simulink model "20240109_HVDCMMCInterconnection"  (R2023b)
settings: Solver=FixedStepDiscrete  StartTime=0.0  StopTime=2  FixedStep=Ts_Power  RelTol=1e-4  EnableMultiTasking=on
PreLoadFcn:
  | HVDCMMCInterconnectionParam
StartFcn:
  | tic
StopFcn:
  | toc
values from neighbouring files (symbols this model uses):
  C_PM = 1.758e-3    (= 0.001758)    [HVDCMMCInterconnectionParam.m]
  Cg = 50e-9    (= 5e-08)    [HVDCMMCInterconnectionParam.m]
  D_R = 0.001    [HVDCMMCInterconnectionParam.m]
  D_Rs = 1e8    (= 100000000)    [HVDCMMCInterconnectionParam.m]
  D_Vf = 0    [HVDCMMCInterconnectionParam.m]
  Fnom = 50    [HVDCMMCInterconnectionParam.m]
  HRM = 2    [HVDCMMCInterconnectionParam.m]
  Ki_Ireg = 6    [HVDCMMCInterconnectionParam.m]
  Ki_Preg = 1.0    (= 1)    [HVDCMMCInterconnectionParam.m]
  Ki_Qreg = 1.0    (= 1)    [HVDCMMCInterconnectionParam.m]
  Ki_VDCreg = 100    [HVDCMMCInterconnectionParam.m]
  Kp_Ireg = 0.6    [HVDCMMCInterconnectionParam.m]
  Kp_Preg = 0.5/3    (= 0.166666666667)    [HVDCMMCInterconnectionParam.m]
  Kp_Qreg = 0.5/3    (= 0.166666666667)    [HVDCMMCInterconnectionParam.m]
  Kp_VDCreg = 4    [HVDCMMCInterconnectionParam.m]
  L_cable = 15e-3    (= 0.015)    [HVDCMMCInterconnectionParam.m]
  Larm = Larm_pu*(Zb_ac/(2*pi*Fnom))    [HVDCMMCInterconnectionParam.m]
  Lff = Larm_pu/2    (= 0.075)    [HVDCMMCInterconnectionParam.m]
  Limits_Ireg = [ 2.0  -2.0]    [HVDCMMCInterconnectionParam.m]
  Limits_Preg = [ 1.2, 0.8 ]    [HVDCMMCInterconnectionParam.m]
  Limits_Qreg = [ 0.25, -0.25 ]    [HVDCMMCInterconnectionParam.m]
  Limits_VDCreg = [ 2.0  -2.0]    [HVDCMMCInterconnectionParam.m]
  Lxfo = 0.12    [HVDCMMCInterconnectionParam.m]
  Nb_PM = 36    [HVDCMMCInterconnectionParam.m]
  Pnom = 1000e6    (= 1000000000)    [HVDCMMCInterconnectionParam.m]
  R_cable = 0.5    [HVDCMMCInterconnectionParam.m]
  R_startup = 400    [HVDCMMCInterconnectionParam.m]
  Rarm = Rarm_pu*Zb_ac    [HVDCMMCInterconnectionParam.m]
  Rff = Rarm_pu/2    (= 0.00075)    [HVDCMMCInterconnectionParam.m]
  Rg = 100    [HVDCMMCInterconnectionParam.m]
  Rxfo = 0.003    [HVDCMMCInterconnectionParam.m]
  Slope_Pref = 0.5    [HVDCMMCInterconnectionParam.m]
  Slope_Qref = 0.5    [HVDCMMCInterconnectionParam.m]
  Slope_Vdc_ref = Vnom_dc/5    (= 128000)    [HVDCMMCInterconnectionParam.m]
  Tbrk1_On = 0.1    [HVDCMMCInterconnectionParam.m]
  Tbrk2_On = 1.0    (= 1)    [HVDCMMCInterconnectionParam.m]
  Tdeblock = 1.5    [HVDCMMCInterconnectionParam.m]
  Tfault = 9999    [HVDCMMCInterconnectionParam.m]
  Ton_Converter2 = 4    [HVDCMMCInterconnectionParam.m]
  Ton_PQreg = 4    [HVDCMMCInterconnectionParam.m]
  Ton_VDCreg = 1.5    [HVDCMMCInterconnectionParam.m]
  Ts = Ts_Control    (= 4e-05)    [HVDCMMCInterconnectionParam.m]
  Ts_Control = 40e-6    (= 4e-05)    [HVDCMMCInterconnectionParam.m]
  Ts_Power = 20e-6    (= 2e-05)    [HVDCMMCInterconnectionParam.m]
  Vb_ac = sqrt(2/3)*Vnom_sec    [HVDCMMCInterconnectionParam.m]
  Vb_dc = Vnom_dc    (= 640000)    [HVDCMMCInterconnectionParam.m]
  Vc0_PM = 0    [HVDCMMCInterconnectionParam.m]
  Vnom_dc = 640e3    (= 640000)    [HVDCMMCInterconnectionParam.m]
  Vnom_prim = 400e3    (= 400000)    [HVDCMMCInterconnectionParam.m]
  Vnom_sec = 333e3    (= 333000)    [HVDCMMCInterconnectionParam.m]
  w = 2*pi*Fnom    (= 314.159265359)    [HVDCMMCInterconnectionParam.m]
undefined symbols (not defined in the file or in its folder): DiscIntNeverNeededParam, gcbh, Pcc, S, sps_AC, sps_ACDC2, sps_rtmsupport
libraries: simulink x48, spsControlledVoltageSourceLib x30, spsCurrentMeasurementLib x30, MMC_Lib x30, spsDiodeLib x20, spsSeriesRLCBranchLib x14, powerlib_extras x12, spsVoltageMeasurementLib x12, spsSecondOrderFilterLib x8, spsabctodq0Lib x8, spsGroundLib x7, spsMeanLib x4
(part 8 of 9)

== system 20240109_HVDCMMCInterconnection/MMC/Half-Bridge MMC Ap (Aggregate model of 36 PM)7 ==
  Uref : Inport
  Controlled Voltage Source : spsControlledVoltageSourceLib/Controlled Voltage Source  Initialize=on  Source_Type=AC  Amplitude=0  Phase=0  Frequency=0  Measurements=None
  Controlled Voltage Source1 : spsControlledVoltageSourceLib/Controlled Voltage Source  Initialize=on  Source_Type=AC  Amplitude=0  Phase=0  Frequency=0  Measurements=None
  Current Measurement : spsCurrentMeasurementLib/Current Measurement  PhasorSimulation=off  OutputType=Complex  PSBequivalent=0
  Current Measurement1 : spsCurrentMeasurementLib/Current Measurement  PhasorSimulation=off  OutputType=Complex  PSBequivalent=0
  Demux : Demux  Outputs=2
  Diode : spsDiodeLib/Diode  Ron=Ron_Diode  Lon=0  Vf=Vf_Diode  IC=0  UseSnubber=0  Rs=Rs_Diode  Cs=Cs_Diode  Measurements=off
  Diode1 : spsDiodeLib/Diode  Ron=Ron_Diode  Lon=0  Vf=Vf_Diode  IC=0  UseSnubber=0  Rs=Rs_Diode  Cs=Cs_Diode  Measurements=off
  Discrete-Time Integrator1 : DiscreteIntegrator  IntegratorMethod=Integration: Trapezoidal  gainval=1  InitialCondition=Vc_Initial  SampleTime=Ts  UpperSaturationLimit=5000  LowerSaturationLimit=500  ICPrevOutput=DiscIntNeverNeededParam  ICPrevScaledInput=DiscIntNeverNeededParam
  Gain1 : Gain  Gain=n
  Gain4 : Gain  Gain=1/(C*n)
  Gain5 : Gain  Gain=2
  Mux1 : Mux  Inputs=2
  Product3 : Product
  Product4 : Product
  Scope : Scope  NumInputPorts=3
  Sum3 : Sum  Inputs=1  InputSameDT=on  SaturateOnIntegerOverflow=on  OutDataTypeStr=Inherit: Same as first input
  Sum4 : Sum  Inputs=+-  InputSameDT=on  SaturateOnIntegerOverflow=on  OutDataTypeStr=Inherit: Same as first input
  Unit Delay2 : UnitDelay  SampleTime=Ts  HasFrameUpgradeWarning=on
  Unit Delay5 : UnitDelay  InitialCondition=Vc_Initial  SampleTime=Ts  HasFrameUpgradeWarning=on
  Unit Delay6 : UnitDelay  InitialCondition=Vc_Initial  SampleTime=Ts  HasFrameUpgradeWarning=on
  Voltage Measurement : spsVoltageMeasurementLib/Voltage Measurement  PhasorSimulation=off  OutputType=Complex  PSBequivalent=0
  1 : PMIOPort  Side=Left
  2 : PMIOPort  Port=2  Side=Left
  Vc : Outport  VectorParamsAs1DForOutWhenUnconnected=off
  wires:
  Demux/1 -> Scope/1, [Vin]
  [Vin] -> Controlled Voltage Source/1
  Current Measurement1/1 -> [Icap]
  Product3/1 -> Sum3/1
  Demux/2 -> Scope/2, [Vbl]
  [Imod] -> Mux1/1
  Sum3/1 -> Gain4/1
  Unit Delay5/1 -> Sum4/2
  Gain5/1 -> Sum4/1
  Mux1/1 -> Unit Delay2/1
  Uref/1 -> Gain1/1
  Sum4/1 -> Vc/1, Product4/2
  Current Measurement/1 -> [Imod]
  Unit Delay2/1 -> Product3/2
  Discrete-Time Integrator1/1 -> Unit Delay6/1
  Product4/1 -> Demux/1
  [Vbl] -> Controlled Voltage Source1/1
  [Icap] -> Mux1/2
  Gain4/1 -> Discrete-Time Integrator1/1
  Unit Delay6/1 -> Gain5/1, Unit Delay5/1
  Gain1/1 -> Product3/1, Product4/1
  Voltage Measurement/1 -> [Vsm]
  [Vsm] -> Scope/3
  connections:
  Diode1/LConn1 -- Current Measurement/RConn1 -- Diode/RConn1
  Controlled Voltage Source1/LConn1 -- Diode/LConn1 -- 2/RConn1 -- Voltage Measurement/LConn2
  Controlled Voltage Source1/RConn1 -- Current Measurement1/RConn1
  Diode1/RConn1 -- Current Measurement1/LConn1
  Controlled Voltage Source/RConn1 -- 1/RConn1 -- Voltage Measurement/LConn1
  Controlled Voltage Source/LConn1 -- Current Measurement/LConn1

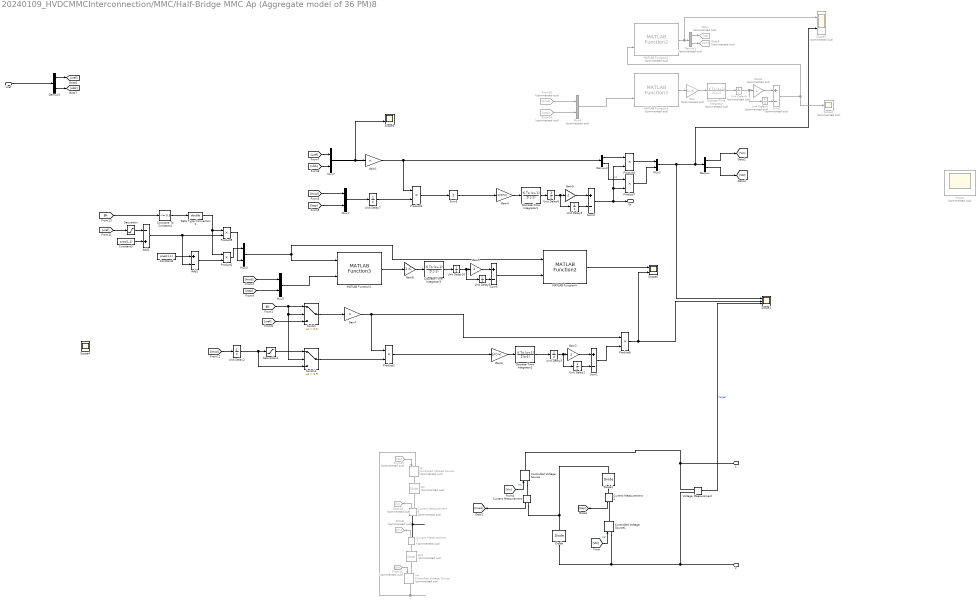
== system 20240109_HVDCMMCInterconnection/MMC/Half-Bridge MMC Ap (Aggregate model of 36 PM)8 ==
  Uref : Inport
  Add1 : Sum  Inputs=+-
  Add2 : Sum  Inputs=-+
  Compare To Constant1 : simulink/Logic and Bit Operations/Compare To Constant  relop=<=  const=0.5  OutDataTypeStr=boolean
  Constant3 : Constant  Value=ones(1,1)
  Constant4 : Constant  Value=ones(1,1)
  Controlled Voltage Source : spsControlledVoltageSourceLib/Controlled Voltage Source  Initialize=on  Source_Type=AC  Amplitude=0  Phase=0  Frequency=0  Measurements=None
  Controlled Voltage Source1 : spsControlledVoltageSourceLib/Controlled Voltage Source  Initialize=on  Source_Type=AC  Amplitude=0  Phase=0  Frequency=0  Measurements=None
  Current Measurement : spsCurrentMeasurementLib/Current Measurement  PhasorSimulation=off  OutputType=Complex  PSBequivalent=0
  Current Measurement1 : spsCurrentMeasurementLib/Current Measurement  PhasorSimulation=off  OutputType=Complex  PSBequivalent=0
  Current Measurement7 : spsCurrentMeasurementLib/Current Measurement  Commented=on  PhasorSimulation=off  OutputType=Complex  PSBequivalent=0
  Current Measurement8 : spsCurrentMeasurementLib/Current Measurement  Commented=on  PhasorSimulation=off  OutputType=Complex  PSBequivalent=0
  Data Type Conversion2 : DataTypeConversion  OutDataTypeStr=double  SaturateOnIntegerOverflow=off  RndMeth=Floor
  Demux : Demux  Outputs=2
  Demux1 : Demux  Commented=on  Outputs=2
  Demux2 : Demux  Outputs=2
  Demux5 : Demux  Outputs=2
  Diode : spsDiodeLib/Diode  Ron=0.0001  Lon=0  Vf=0.0001  IC=0  UseSnubber=0  Rs=1e9  Cs=Cs_Diode  Measurements=off
  Diode1 : spsDiodeLib/Diode  Ron=0.0001  Lon=0  Vf=0.0001  IC=0  UseSnubber=0  Rs=1e9  Cs=Cs_Diode  Measurements=off
  Discrete-Time Integrator : DiscreteIntegrator  Commented=on  IntegratorMethod=Integration: Trapezoidal  gainval=1  InitialCondition=Vc_Initial  SampleTime=Ts  UpperSaturationLimit=5000  LowerSaturationLimit=500  ICPrevOutput=DiscIntNeverNeededParam  ICPrevScaledInput=DiscIntNeverNeededParam
  Discrete-Time Integrator1 : DiscreteIntegrator  IntegratorMethod=Integration: Trapezoidal  gainval=1  InitialCondition=Vc_Initial  SampleTime=Ts  UpperSaturationLimit=5000  LowerSaturationLimit=500  ICPrevOutput=DiscIntNeverNeededParam  ICPrevScaledInput=DiscIntNeverNeededParam
  Discrete-Time Integrator2 : DiscreteIntegrator  IntegratorMethod=Integration: Trapezoidal  gainval=1  InitialCondition=Vc_Initial  SampleTime=Ts  UpperSaturationLimit=5000  LowerSaturationLimit=500  ICPrevOutput=DiscIntNeverNeededParam  ICPrevScaledInput=DiscIntNeverNeededParam
  Discrete-Time Integrator3 : DiscreteIntegrator  IntegratorMethod=Integration: Trapezoidal  gainval=1  InitialCondition=Vc_Initial  SampleTime=Ts  UpperSaturationLimit=5000  LowerSaturationLimit=500  ICPrevOutput=DiscIntNeverNeededParam  ICPrevScaledInput=DiscIntNeverNeededParam
  Dp : spsDiodeLib/Diode  Commented=on  Ron=Ron_Diode  Lon=0  Vf=Vf_Diode  IC=0  UseSnubber=off  Rs=Rs_Diode  Cs=Cs_Diode  Measurements=off
  Dp1 : spsDiodeLib/Diode  Commented=on  Ron=Ron_Diode  Lon=0  Vf=Vf_Diode  IC=0  UseSnubber=off  Rs=Rs_Diode  Cs=Cs_Diode  Measurements=off
  From10 : From  Commented=on  GotoTag=Imod
  From14 : From  Commented=on  GotoTag=Icap
  From15 : From  Commented=on  GotoTag=Vp
  From16 : From  Commented=on  GotoTag=Vm
  Gain : Gain  Commented=on  Gain=-1./C
  Gain1 : Gain  Gain=n
  Gain2 : Gain  Gain=2
  Gain3 : Gain  Gain=1/(C*n)
  Gain4 : Gain  Gain=1/(C*n)
  Gain5 : Gain  Gain=2
  Gain6 : Gain  Gain=-1./C
  Gain7 : Gain  Gain=n
  Gain8 : Gain  Commented=on  Gain=2
  Gain9 : Gain  Gain=2
  Goto : Goto  Commented=on  GotoTag=Vp
  Goto18 : Goto  Commented=on  GotoTag=Ip
  Goto5 : Goto  Commented=on  GotoTag=Vm
  Goto8 : Goto  Commented=on  GotoTag=Im
  MATLAB Function1 : spsHalfBridgeMMCmodel/AVG Discrete/MATLAB Function3  n=1  ModelType=3
  MATLAB Function2 : spsHalfBridgeMMCmodel/AVG Discrete/MATLAB Function2  Commented=on  n=1  ModelType=3
  MATLAB Function3 : spsHalfBridgeMMCmodel/AVG Discrete/MATLAB Function3  Commented=on  n=1  ModelType=3
  MATLAB Function4 : spsHalfBridgeMMCmodel/AVG Discrete/MATLAB Function2  n=1  ModelType=3
  Mux{1..3,5,7} (5 alike) : Mux  Inputs=2
  Mux4 : Mux  Commented=on  Inputs=2
  Product{1..5,7..8} (7 alike) : Product
  Saturation : Saturate  UpperLimit=1  LowerLimit=-1
  Saturation2 : Saturate  UpperLimit=inf  LowerLimit=0
  Scope : Scope  Commented=on  NumInputPorts=2
  Scope1 : Scope  NumInputPorts=3
  Scope2 : Scope  Commented=on
  Scope3 : Scope  Commented=on  NumInputPorts=2
  Scope4 : Scope  NumInputPorts=2
  Scope5 : Scope  NumInputPorts=2
  Scope6 : Scope  NumInputPorts=2
  Sum1 : Sum  Inputs=+-  InputSameDT=on  SaturateOnIntegerOverflow=on  OutDataTypeStr=Inherit: Same as first input
  Sum2 : Sum  Commented=on  Inputs=+-  InputSameDT=on  SaturateOnIntegerOverflow=on  OutDataTypeStr=Inherit: Same as first input
  Sum3 : Sum  Inputs=1  InputSameDT=on  SaturateOnIntegerOverflow=on  OutDataTypeStr=Inherit: Same as first input
  Sum4 : Sum  Inputs=+-  InputSameDT=on  SaturateOnIntegerOverflow=on  OutDataTypeStr=Inherit: Same as first input
  Sum5 : Sum  Inputs=+-  InputSameDT=on  SaturateOnIntegerOverflow=on  OutDataTypeStr=Inherit: Same as first input
  Switch : Switch  Criteria=u2 > Threshold  Threshold=0.5  SaturateOnIntegerOverflow=off  InputSameDT=off
  Switch1 : Switch  Criteria=u2 > Threshold  Threshold=0.5  SaturateOnIntegerOverflow=off  InputSameDT=off
  Unit Delay{1,3,5..6,9..10} (6 alike) : UnitDelay  InitialCondition=Vc_Initial  SampleTime=Ts  HasFrameUpgradeWarning=on
  Unit Delay2 : UnitDelay  SampleTime=Ts  HasFrameUpgradeWarning=on
  Unit Delay4 : UnitDelay  Commented=on  InitialCondition=Vc_Initial  SampleTime=Ts  HasFrameUpgradeWarning=on
  Unit Delay7 : UnitDelay  SampleTime=Ts  HasFrameUpgradeWarning=on
  Unit Delay8 : UnitDelay  Commented=on  InitialCondition=Vc_Initial  SampleTime=Ts  HasFrameUpgradeWarning=on
  Vm : spsControlledVoltageSourceLib/Controlled Voltage Source  Commented=on  Initialize=off  Source_Type=AC  Amplitude=0  Phase=0  Frequency=0  Measurements=None
  Voltage Measurement : spsVoltageMeasurementLib/Voltage Measurement  PhasorSimulation=off  OutputType=Complex  PSBequivalent=0
  Vp : spsControlledVoltageSourceLib/Controlled Voltage Source  Commented=on  Initialize=off  Source_Type=AC  Amplitude=0  Phase=0  Frequency=0  Measurements=None
  1 : PMIOPort  Side=Left
  2 : PMIOPort  Port=2  Side=Left
  Vc : Outport  VectorParamsAs1DForOutWhenUnconnected=off
  wires:
  Demux/1 -> [Vin]
  [Vin] -> Controlled Voltage Source/1  "Vin"
  Product3/1 -> Sum3/1
  Demux/2 -> [Vbl]
  [Imod] -> Mux1/1
  Unit Delay5/1 -> Sum4/2
  Gain5/1 -> Sum4/1
  Sum4/1 -> Product7/2, Product4/2, Vc/1  "Vc"
  Discrete-Time Integrator1/1 -> Unit Delay6/1
  Mux2/1 -> Scope1/1, Scope3/2, Demux/1
  [Vbl] -> Controlled Voltage Source1/1  "Vbl"
  [Icap] -> Mux1/2
  Gain4/1 -> Discrete-Time Integrator1/1
  Unit Delay6/1 -> Gain5/1, Unit Delay5/1
  Mux1/1 -> Unit Delay7/1
  Mux7/1 -> Scope5/2, Gain1/1
  Gain3/1 -> Discrete-Time Integrator2/1
  Demux2/1 -> Product4/1
  Demux2/2 -> Product7/1
  Product4/1 -> Mux2/1
  Product7/1 -> Mux2/2
  Unit Delay3/1 -> Gain2/1, Unit Delay1/1
  Unit Delay1/1 -> Sum1/2
  Gain2/1 -> Sum1/1
  Discrete-Time Integrator2/1 -> Unit Delay3/1
  Product2/1 -> Gain3/1
  Sum1/1 -> Product8/2
  Demux5/2 -> [ublk]
  [uref] -> Mux7/1
  [ublk] -> Mux7/2
  Current Measurement/1 -> [Imod]
  Current Measurement1/1 -> [Icap]
  Unit Delay7/1 -> Product3/2
  [uref] -> Switch/3
  [Imod] -> Unit Delay2/1
  Saturation2/1 -> Switch1/1
  [Blk] -> Switch1/2, Switch/2, Switch/1
  Switch1/1 -> Product2/2
  Product8/1 -> Scope6/2, Scope1/2
  Unit Delay2/1 -> Saturation2/1, Switch1/3
  Gain1/1 -> Demux2/1, Product3/1
  Gain7/1 -> Product2/1, Product8/1
  Demux5/1 -> [uref]
  Uref/1 -> Demux5/1
  Voltage Measurement/1 -> Scope1/3  "Target"
  Gain8/1 -> Sum2/1
  Data Type Conversion2/1 -> Product5/1, Product1/1
  [Blk] -> Compare To Constant1/1
  Unit Delay4/1 -> Sum2/2
  Unit Delay8/1 -> Unit Delay4/1, Gain8/1
  Gain/1 -> Discrete-Time Integrator/1
  MATLAB Function2/1 -> Scope3/1, Demux1/1
  Add2/1 -> Add1/2, Product5/2
  MATLAB Function3/1 -> Gain/1
  Constant4/1 -> Add1/1
  Demux1/1 -> Goto/1
  [uref] -> Saturation/1
  Compare To Constant1/1 -> Data Type Conversion2/1
  Sum2/1 -> MATLAB Function2/2, Scope2/1
  Discrete-Time Integrator/1 -> Unit Delay8/1
  Demux1/2 -> Goto5/1
  Add1/1 -> Product1/2
  Product1/1 -> Mux3/1
  Constant3/1 -> Add2/2
  Saturation/1 -> Add2/1
  Sum3/1 -> Gain4/1
  From14/1 -> Mux4/2
  From10/1 -> Mux4/1
  Mux4/1 -> MATLAB Function3/2
  Product5/1 -> Mux3/2
  Switch/1 -> Gain7/1
  Mux5/1 -> MATLAB Function1/2
  [Imod] -> Mux5/1
  [Icap] -> Mux5/2
  Mux3/1 -> MATLAB Function1/1, MATLAB Function4/1
  Discrete-Time Integrator3/1 -> Unit Delay10/1
  Gain6/1 -> Discrete-Time Integrator3/1
  MATLAB Function1/1 -> Gain6/1
  Gain9/1 -> Sum5/1
  Unit Delay9/1 -> Sum5/2
  Unit Delay10/1 -> Unit Delay9/1, Gain9/1
  Sum5/1 -> MATLAB Function4/2
  MATLAB Function4/1 -> Scope6/1
  Current Measurement8/1 -> Goto18/1
  From16/1 -> Vm/1
  From15/1 -> Vp/1
  Current Measurement7/1 -> Goto8/1
  connections:
  Current Measurement/RConn1 -- Diode1/LConn1 -- Diode/RConn1
  Diode/LConn1 -- Voltage Measurement/LConn2 -- 2/RConn1 -- Controlled Voltage Source1/LConn1
  Controlled Voltage Source1/RConn1 -- Current Measurement1/RConn1
  Diode1/RConn1 -- Current Measurement1/LConn1
  1/RConn1 -- Voltage Measurement/LConn1 -- Controlled Voltage Source/RConn1
  Controlled Voltage Source/LConn1 -- Current Measurement/LConn1
  Vm/RConn1 -- Vp/LConn1
  Current Measurement8/LConn1 -- Current Measurement7/RConn1
  Vp/RConn1 -- Dp/RConn1
  Dp1/LConn1 -- Vm/LConn1
  Dp1/RConn1 -- Current Measurement7/LConn1
  Current Measurement8/RConn1 -- Dp/LConn1

== system 20240109_HVDCMMCInterconnection/MMC/Meas_An ==
  An_I : spsCurrentMeasurementLib/Current Measurement  PhasorSimulation=off  OutputType=Complex  PSBequivalent=0
  An_V : spsVoltageMeasurementLib/Voltage Measurement  PhasorSimulation=off  OutputType=Complex  PSBequivalent=0
  I1 : PMIOPort  Side=Left
  I2 : PMIOPort  Port=2  Side=Left
  O1 : PMIOPort  Port=3  Side=Right
  O2 : PMIOPort  Port=4  Side=Right
  tag scope: I_Am=global, V12_Am=global
  wires:
  An_V/1 -> [V12_Am]
  An_I/1 -> [I_Am]
  connections:
  An_V/LConn2 -- O2/RConn1 -- I2/RConn1
  An_I/LConn1 -- O1/RConn1
  An_V/LConn1 -- An_I/RConn1 -- I1/RConn1

== system 20240109_HVDCMMCInterconnection/MMC/Meas_Ap ==
  Ap_I : spsCurrentMeasurementLib/Current Measurement  PhasorSimulation=off  OutputType=Complex  PSBequivalent=0
  Ap_V : spsVoltageMeasurementLib/Voltage Measurement  PhasorSimulation=off  OutputType=Complex  PSBequivalent=0
  I1 : PMIOPort  Side=Left
  I2 : PMIOPort  Port=2  Side=Left
  O1 : PMIOPort  Port=3  Side=Right
  O2 : PMIOPort  Port=4  Side=Right
  tag scope: I_Ap=global, V12_Ap=global
  wires:
  Ap_I/1 -> [I_Ap]
  Ap_V/1 -> [V12_Ap]
  connections:
  Ap_I/RConn1 -- Ap_V/LConn1 -- I1/RConn1
  Ap_I/LConn1 -- O1/RConn1
  I2/RConn1 -- Ap_V/LConn2 -- O2/RConn1

== system 20240109_HVDCMMCInterconnection/MMC/Meas_Bn ==
  Bn_I : spsCurrentMeasurementLib/Current Measurement  PhasorSimulation=off  OutputType=Complex  PSBequivalent=0
  Bn_V : spsVoltageMeasurementLib/Voltage Measurement  PhasorSimulation=off  OutputType=Complex  PSBequivalent=0
  I1 : PMIOPort  Side=Left
  I2 : PMIOPort  Port=2  Side=Left
  O1 : PMIOPort  Port=3  Side=Right
  O2 : PMIOPort  Port=4  Side=Right
  tag scope: I_Bm=global, V12_Bm=global
  wires:
  Bn_I/1 -> [I_Bm]
  Bn_V/1 -> [V12_Bm]
  connections:
  I1/RConn1 -- Bn_I/RConn1 -- Bn_V/LConn1
  Bn_I/LConn1 -- O1/RConn1
  I2/RConn1 -- O2/RConn1 -- Bn_V/LConn2

== system 20240109_HVDCMMCInterconnection/MMC/Meas_Bp ==
  Bp_I : spsCurrentMeasurementLib/Current Measurement  PhasorSimulation=off  OutputType=Complex  PSBequivalent=0
  Bp_V : spsVoltageMeasurementLib/Voltage Measurement  PhasorSimulation=off  OutputType=Complex  PSBequivalent=0
  I1 : PMIOPort  Side=Left
  I2 : PMIOPort  Port=2  Side=Left
  O1 : PMIOPort  Port=3  Side=Right
  O2 : PMIOPort  Port=4  Side=Right
  tag scope: I_Bp=global, V12_Bp=global
  wires:
  Bp_V/1 -> [V12_Bp]
  Bp_I/1 -> [I_Bp]
  connections:
  Bp_V/LConn2 -- O2/RConn1 -- I2/RConn1
  Bp_I/LConn1 -- O1/RConn1
  Bp_V/LConn1 -- Bp_I/RConn1 -- I1/RConn1

== system 20240109_HVDCMMCInterconnection/MMC/Meas_Cn ==
  Cn_I : spsCurrentMeasurementLib/Current Measurement  PhasorSimulation=off  OutputType=Complex  PSBequivalent=0
  Cn_V : spsVoltageMeasurementLib/Voltage Measurement  PhasorSimulation=off  OutputType=Complex  PSBequivalent=0
  I1 : PMIOPort  Side=Left
  I2 : PMIOPort  Port=2  Side=Left
  O1 : PMIOPort  Port=3  Side=Right
  O2 : PMIOPort  Port=4  Side=Right
  tag scope: I_Cm=global, V12_Cm=global
  wires:
  Cn_V/1 -> [V12_Cm]
  Cn_I/1 -> [I_Cm]
  connections:
  Cn_V/LConn2 -- O2/RConn1 -- I2/RConn1
  Cn_I/LConn1 -- O1/RConn1
  Cn_V/LConn1 -- Cn_I/RConn1 -- I1/RConn1

== system 20240109_HVDCMMCInterconnection/MMC/Meas_Cp ==
  Cp_I : spsCurrentMeasurementLib/Current Measurement  PhasorSimulation=off  OutputType=Complex  PSBequivalent=0
  Cp_V : spsVoltageMeasurementLib/Voltage Measurement  PhasorSimulation=off  OutputType=Complex  PSBequivalent=0
  I1 : PMIOPort  Side=Left
  I2 : PMIOPort  Port=2  Side=Left
  O1 : PMIOPort  Port=3  Side=Right
  O2 : PMIOPort  Port=4  Side=Right
  tag scope: I_Cp=global, V12_Cp=global
  wires:
  Cp_I/1 -> [I_Cp]
  Cp_V/1 -> [V12_Cp]
  connections:
  I1/RConn1 -- Cp_I/RConn1 -- Cp_V/LConn1
  Cp_I/LConn1 -- O1/RConn1
  I2/RConn1 -- O2/RConn1 -- Cp_V/LConn2

== system 20240109_HVDCMMCInterconnection/MMC/Uref2m2 ==
  Uref_ABC : Inport  PortDimensions=3
  Block : Inport  Port=2
  Add1 : Sum
  Add2 : Sum
  Compare To Constant{1..4} (4 alike) : simulink/Logic and Bit Operations/Compare To Constant  relop=<=  const=0.5  OutDataTypeStr=boolean
  Constant1 : Constant
  Constant2 : Constant  Value=[0 0 0]
  Constant3 : Constant  Value=[1 1 1]
  Constant6 : Constant
  Constant7 : Constant  Value=[0 0 0]
  Constant9 : Constant  Value=[1 1 1]
  Demux{,2..4} (4 alike) : Demux  Outputs=3
  Gain1 : Gain  Gain=-1
  Gain2 : Gain  Gain=0.5
  Gain3 : Gain  Gain=0.5
  Mux{,1..2,4..6} (6 alike) : Mux  Inputs=2
  Saturation{1,3..5} (4 alike) : Saturate  UpperLimit=1  LowerLimit=0
  Switch{1..4} (4 alike) : Switch  Criteria=u2 ~= 0  SaturateOnIntegerOverflow=off  InputSameDT=off
  Uref_Ap : Outport
  Uref_Bp : Outport  Port=2
  Uref_Cp : Outport  Port=3
  Uref_An : Outport  Port=4
  Uref_Bn : Outport  Port=5
  Uref_Cn : Outport  Port=6
  wires:
  Add1/1 -> Gain3/1
  Gain3/1 -> Switch1/1
  Constant7/1 -> Switch1/3, Switch2/1
  Compare To Constant1/1 -> Switch2/2
  Constant6/1 -> Add1/2
  Constant9/1 -> Switch2/3
  Compare To Constant2/1 -> Switch1/2
  Gain1/1 -> Add1/1
  Mux/1 -> Uref_Ap/1
  Switch1/1 -> Saturation1/1
  Switch2/1 -> Saturation3/1
  Demux/1 -> Mux/1
  Demux2/1 -> Mux/2
  Demux/2 -> Mux1/1
  Demux2/2 -> Mux1/2
  Demux2/3 -> Mux2/2
  Demux/3 -> Mux2/1
  Demux4/1 -> Mux4/2
  Demux4/2 -> Mux5/2
  Constant1/1 -> Add2/2
  Compare To Constant4/1 -> Switch3/2
  Compare To Constant3/1 -> Switch4/2
  Add2/1 -> Gain2/1
  Constant2/1 -> Switch3/3, Switch4/1
  Block/1 -> Compare To Constant1/1, Compare To Constant4/1, Compare To Constant3/1, Compare To Constant2/1
  Uref_ABC/1 -> Add2/1, Gain1/1
  Switch3/1 -> Saturation4/1
  Demux3/2 -> Mux5/1
  Demux3/3 -> Mux6/1
  Constant3/1 -> Switch4/3
  Demux3/1 -> Mux4/1
  Switch4/1 -> Saturation5/1
  Gain2/1 -> Switch3/1
  Demux4/3 -> Mux6/2
  Saturation1/1 -> Demux/1
  Saturation3/1 -> Demux2/1
  Saturation4/1 -> Demux3/1
  Saturation5/1 -> Demux4/1
  Mux1/1 -> Uref_Bp/1
  Mux2/1 -> Uref_Cp/1
  Mux4/1 -> Uref_An/1
  Mux5/1 -> Uref_Bn/1
  Mux6/1 -> Uref_Cn/1

== system 20240109_HVDCMMCInterconnection/Sources/3ph SM1 ==
  Uref_An : Inport
  An_Ipos : Inport  Port=2
  An_Icap : Inport  Port=3
  Demux : Demux  Outputs=2
  Demux2 : Demux  Outputs=2
  Discrete-Time Integrator1 : DiscreteIntegrator  IntegratorMethod=Integration: Trapezoidal  gainval=1  SampleTime=Ts_Power  UpperSaturationLimit=5000  LowerSaturationLimit=500  ICPrevOutput=DiscIntNeverNeededParam  ICPrevScaledInput=DiscIntNeverNeededParam
  Gain1 : Gain  Gain=Nb_PM
  Gain4 : Gain  Gain=1/(C_PM*Nb_PM)
  Gain5 : Gain  Gain=2
  Mux1 : Mux  Inputs=2
  Mux2 : Mux  Inputs=2
  Product3 : Product
  Product4 : Product
  Product7 : Product
  Sum3 : Sum  Inputs=1  InputSameDT=on  SaturateOnIntegerOverflow=on  OutDataTypeStr=Inherit: Same as first input
  Sum4 : Sum  Inputs=+-  InputSameDT=on  SaturateOnIntegerOverflow=on  OutDataTypeStr=Inherit: Same as first input
  Unit Delay5 : UnitDelay  SampleTime=Ts_Power  HasFrameUpgradeWarning=on
  Unit Delay6 : UnitDelay  SampleTime=Ts_Power  HasFrameUpgradeWarning=on
  Unit Delay7 : UnitDelay  SampleTime=Ts_Power  HasFrameUpgradeWarning=on
  An_Vbl : Outport
  An_Vin : Outport  Port=2
  wires:
  Gain5/1 -> Sum4/1
  Gain1/1 -> Demux2/1, Product3/1
  Mux2/1 -> Demux/1
  Demux/1 -> An_Vin/1
  Uref_An/1 -> Gain1/1
  Gain4/1 -> Discrete-Time Integrator1/1
  Mux1/1 -> Unit Delay7/1
  Demux2/2 -> Product7/1
  Unit Delay6/1 -> Gain5/1, Unit Delay5/1
  An_Icap/1 -> Mux1/2
  Demux2/1 -> Product4/1
  Discrete-Time Integrator1/1 -> Unit Delay6/1
  Sum4/1 -> Product7/2, Product4/2  "Vc"
  Unit Delay5/1 -> Sum4/2
  Sum3/1 -> Gain4/1
  Product3/1 -> Sum3/1
  Product4/1 -> Mux2/1  "Vin"
  Demux/2 -> An_Vbl/1
  Product7/1 -> Mux2/2  "Vbl"
  Unit Delay7/1 -> Product3/2
  An_Ipos/1 -> Mux1/1

== system 20240109_HVDCMMCInterconnection/Sources/3ph SM2 ==
  Uref_An : Inport
  An_Ipos : Inport  Port=2
  An_Icap : Inport  Port=3
  Demux : Demux  Outputs=2
  Demux2 : Demux  Outputs=2
  Discrete-Time Integrator1 : DiscreteIntegrator  IntegratorMethod=Integration: Trapezoidal  gainval=1  SampleTime=Ts_Power  UpperSaturationLimit=5000  LowerSaturationLimit=500  ICPrevOutput=DiscIntNeverNeededParam  ICPrevScaledInput=DiscIntNeverNeededParam
  Gain1 : Gain  Gain=Nb_PM
  Gain4 : Gain  Gain=1/(C_PM*Nb_PM)
  Gain5 : Gain  Gain=2
  Mux1 : Mux  Inputs=2
  Mux2 : Mux  Inputs=2
  Product3 : Product
  Product4 : Product
  Product7 : Product
  Sum3 : Sum  Inputs=1  InputSameDT=on  SaturateOnIntegerOverflow=on  OutDataTypeStr=Inherit: Same as first input
  Sum4 : Sum  Inputs=+-  InputSameDT=on  SaturateOnIntegerOverflow=on  OutDataTypeStr=Inherit: Same as first input
  Unit Delay5 : UnitDelay  SampleTime=Ts_Power  HasFrameUpgradeWarning=on
  Unit Delay6 : UnitDelay  SampleTime=Ts_Power  HasFrameUpgradeWarning=on
  Unit Delay7 : UnitDelay  SampleTime=Ts_Power  HasFrameUpgradeWarning=on
  An_Vbl : Outport
  An_Vin : Outport  Port=2
  wires:
  Gain5/1 -> Sum4/1
  Gain1/1 -> Demux2/1, Product3/1
  Mux2/1 -> Demux/1
  Demux/1 -> An_Vin/1
  Uref_An/1 -> Gain1/1
  Gain4/1 -> Discrete-Time Integrator1/1
  Mux1/1 -> Unit Delay7/1
  Demux2/2 -> Product7/1
  Unit Delay6/1 -> Gain5/1, Unit Delay5/1
  An_Icap/1 -> Mux1/2
  Demux2/1 -> Product4/1
  Discrete-Time Integrator1/1 -> Unit Delay6/1
  Sum4/1 -> Product7/2, Product4/2  "Vc"
  Unit Delay5/1 -> Sum4/2
  Sum3/1 -> Gain4/1
  Product3/1 -> Sum3/1
  Product4/1 -> Mux2/1  "Vin"
  Demux/2 -> An_Vbl/1
  Product7/1 -> Mux2/2  "Vbl"
  Unit Delay7/1 -> Product3/2
  An_Ipos/1 -> Mux1/1

== system 20240109_HVDCMMCInterconnection/Sources/3ph SM3 ==
  Uref_An : Inport
  An_Ipos : Inport  Port=2
  An_Icap : Inport  Port=3
  Demux : Demux  Outputs=2
  Demux2 : Demux  Outputs=2
  Discrete-Time Integrator1 : DiscreteIntegrator  IntegratorMethod=Integration: Trapezoidal  gainval=1  SampleTime=Ts_Power  UpperSaturationLimit=5000  LowerSaturationLimit=500  ICPrevOutput=DiscIntNeverNeededParam  ICPrevScaledInput=DiscIntNeverNeededParam
  Gain1 : Gain  Gain=Nb_PM
  Gain4 : Gain  Gain=1/(C_PM*Nb_PM)
  Gain5 : Gain  Gain=2
  Mux1 : Mux  Inputs=2
  Mux2 : Mux  Inputs=2
  Product3 : Product
  Product4 : Product
  Product7 : Product
  Sum3 : Sum  Inputs=1  InputSameDT=on  SaturateOnIntegerOverflow=on  OutDataTypeStr=Inherit: Same as first input
  Sum4 : Sum  Inputs=+-  InputSameDT=on  SaturateOnIntegerOverflow=on  OutDataTypeStr=Inherit: Same as first input
  Unit Delay5 : UnitDelay  SampleTime=Ts_Power  HasFrameUpgradeWarning=on
  Unit Delay6 : UnitDelay  SampleTime=Ts_Power  HasFrameUpgradeWarning=on
  Unit Delay7 : UnitDelay  SampleTime=Ts_Power  HasFrameUpgradeWarning=on
  An_Vbl : Outport
  An_Vin : Outport  Port=2
  wires:
  Gain5/1 -> Sum4/1
  Gain1/1 -> Demux2/1, Product3/1
  Mux2/1 -> Demux/1
  Demux/1 -> An_Vin/1
  Uref_An/1 -> Gain1/1
  Gain4/1 -> Discrete-Time Integrator1/1
  Mux1/1 -> Unit Delay7/1
  Demux2/2 -> Product7/1
  Unit Delay6/1 -> Gain5/1, Unit Delay5/1
  An_Icap/1 -> Mux1/2
  Demux2/1 -> Product4/1
  Discrete-Time Integrator1/1 -> Unit Delay6/1
  Sum4/1 -> Product7/2, Product4/2  "Vc"
  Unit Delay5/1 -> Sum4/2
  Sum3/1 -> Gain4/1
  Product3/1 -> Sum3/1
  Product4/1 -> Mux2/1  "Vin"
  Demux/2 -> An_Vbl/1
  Product7/1 -> Mux2/2  "Vbl"
  Unit Delay7/1 -> Product3/2
  An_Ipos/1 -> Mux1/1

== system 20240109_HVDCMMCInterconnection/Sources/3ph SM4 ==
  Uref_An : Inport
  An_Ipos : Inport  Port=2
  An_Icap : Inport  Port=3
  Demux : Demux  Outputs=2
  Demux2 : Demux  Outputs=2
  Discrete-Time Integrator1 : DiscreteIntegrator  IntegratorMethod=Integration: Trapezoidal  gainval=1  SampleTime=Ts_Power  UpperSaturationLimit=5000  LowerSaturationLimit=500  ICPrevOutput=DiscIntNeverNeededParam  ICPrevScaledInput=DiscIntNeverNeededParam
  Gain1 : Gain  Gain=Nb_PM
  Gain4 : Gain  Gain=1/(C_PM*Nb_PM)
  Gain5 : Gain  Gain=2
  Mux1 : Mux  Inputs=2
  Mux2 : Mux  Inputs=2
  Product3 : Product
  Product4 : Product
  Product7 : Product
  Sum3 : Sum  Inputs=1  InputSameDT=on  SaturateOnIntegerOverflow=on  OutDataTypeStr=Inherit: Same as first input
  Sum4 : Sum  Inputs=+-  InputSameDT=on  SaturateOnIntegerOverflow=on  OutDataTypeStr=Inherit: Same as first input
  Unit Delay5 : UnitDelay  SampleTime=Ts_Power  HasFrameUpgradeWarning=on
  Unit Delay6 : UnitDelay  SampleTime=Ts_Power  HasFrameUpgradeWarning=on
  Unit Delay7 : UnitDelay  SampleTime=Ts_Power  HasFrameUpgradeWarning=on
  An_Vbl : Outport
  An_Vin : Outport  Port=2
  wires:
  Gain5/1 -> Sum4/1
  Gain1/1 -> Demux2/1, Product3/1
  Mux2/1 -> Demux/1
  Demux/1 -> An_Vin/1
  Uref_An/1 -> Gain1/1
  Gain4/1 -> Discrete-Time Integrator1/1
  Mux1/1 -> Unit Delay7/1
  Demux2/2 -> Product7/1
  Unit Delay6/1 -> Gain5/1, Unit Delay5/1
  An_Icap/1 -> Mux1/2
  Demux2/1 -> Product4/1
  Discrete-Time Integrator1/1 -> Unit Delay6/1
  Sum4/1 -> Product7/2, Product4/2  "Vc"
  Unit Delay5/1 -> Sum4/2
  Sum3/1 -> Gain4/1
  Product3/1 -> Sum3/1
  Product4/1 -> Mux2/1  "Vin"
  Demux/2 -> An_Vbl/1
  Product7/1 -> Mux2/2  "Vbl"
  Unit Delay7/1 -> Product3/2
  An_Ipos/1 -> Mux1/1

== system 20240109_HVDCMMCInterconnection/Sources/3ph SM5 ==
  Uref_An : Inport
  An_Ipos : Inport  Port=2
  An_Icap : Inport  Port=3
  Demux : Demux  Outputs=2
  Demux2 : Demux  Outputs=2
  Discrete-Time Integrator1 : DiscreteIntegrator  IntegratorMethod=Integration: Trapezoidal  gainval=1  SampleTime=Ts_Power  UpperSaturationLimit=5000  LowerSaturationLimit=500  ICPrevOutput=DiscIntNeverNeededParam  ICPrevScaledInput=DiscIntNeverNeededParam
  Gain1 : Gain  Gain=Nb_PM
  Gain4 : Gain  Gain=1/(C_PM*Nb_PM)
  Gain5 : Gain  Gain=2
  Mux1 : Mux  Inputs=2
  Mux2 : Mux  Inputs=2
  Product3 : Product
  Product4 : Product
  Product7 : Product
  Sum3 : Sum  Inputs=1  InputSameDT=on  SaturateOnIntegerOverflow=on  OutDataTypeStr=Inherit: Same as first input
  Sum4 : Sum  Inputs=+-  InputSameDT=on  SaturateOnIntegerOverflow=on  OutDataTypeStr=Inherit: Same as first input
  Unit Delay5 : UnitDelay  SampleTime=Ts_Power  HasFrameUpgradeWarning=on
  Unit Delay6 : UnitDelay  SampleTime=Ts_Power  HasFrameUpgradeWarning=on
  Unit Delay7 : UnitDelay  SampleTime=Ts_Power  HasFrameUpgradeWarning=on
  An_Vbl : Outport
  An_Vin : Outport  Port=2
  wires:
  Gain5/1 -> Sum4/1
  Gain1/1 -> Demux2/1, Product3/1
  Mux2/1 -> Demux/1
  Demux/1 -> An_Vin/1
  Uref_An/1 -> Gain1/1
  Gain4/1 -> Discrete-Time Integrator1/1
  Mux1/1 -> Unit Delay7/1
  Demux2/2 -> Product7/1
  Unit Delay6/1 -> Gain5/1, Unit Delay5/1
  An_Icap/1 -> Mux1/2
  Demux2/1 -> Product4/1
  Discrete-Time Integrator1/1 -> Unit Delay6/1
  Sum4/1 -> Product7/2, Product4/2  "Vc"
  Unit Delay5/1 -> Sum4/2
  Sum3/1 -> Gain4/1
  Product3/1 -> Sum3/1
  Product4/1 -> Mux2/1  "Vin"
  Demux/2 -> An_Vbl/1
  Product7/1 -> Mux2/2  "Vbl"
  Unit Delay7/1 -> Product3/2
  An_Ipos/1 -> Mux1/1

== system 20240109_HVDCMMCInterconnection/Sources/3ph SM6 ==
  Uref_An : Inport
  An_Ipos : Inport  Port=2
  An_Icap : Inport  Port=3
  Demux : Demux  Outputs=2
  Demux2 : Demux  Outputs=2
  Discrete-Time Integrator1 : DiscreteIntegrator  IntegratorMethod=Integration: Trapezoidal  gainval=1  SampleTime=Ts_Power  UpperSaturationLimit=5000  LowerSaturationLimit=500  ICPrevOutput=DiscIntNeverNeededParam  ICPrevScaledInput=DiscIntNeverNeededParam
  Gain1 : Gain  Gain=Nb_PM
  Gain4 : Gain  Gain=1/(C_PM*Nb_PM)
  Gain5 : Gain  Gain=2
  Mux1 : Mux  Inputs=2
  Mux2 : Mux  Inputs=2
  Product3 : Product
  Product4 : Product
  Product7 : Product
  Sum3 : Sum  Inputs=1  InputSameDT=on  SaturateOnIntegerOverflow=on  OutDataTypeStr=Inherit: Same as first input
  Sum4 : Sum  Inputs=+-  InputSameDT=on  SaturateOnIntegerOverflow=on  OutDataTypeStr=Inherit: Same as first input
  Unit Delay5 : UnitDelay  SampleTime=Ts_Power  HasFrameUpgradeWarning=on
  Unit Delay6 : UnitDelay  SampleTime=Ts_Power  HasFrameUpgradeWarning=on
  Unit Delay7 : UnitDelay  SampleTime=Ts_Power  HasFrameUpgradeWarning=on
  An_Vbl : Outport
  An_Vin : Outport  Port=2
  wires:
  Gain5/1 -> Sum4/1
  Gain1/1 -> Demux2/1, Product3/1
  Mux2/1 -> Demux/1
  Demux/1 -> An_Vin/1
  Uref_An/1 -> Gain1/1
  Gain4/1 -> Discrete-Time Integrator1/1
  Mux1/1 -> Unit Delay7/1
  Demux2/2 -> Product7/1
  Unit Delay6/1 -> Gain5/1, Unit Delay5/1
  An_Icap/1 -> Mux1/2
  Demux2/1 -> Product4/1
  Discrete-Time Integrator1/1 -> Unit Delay6/1
  Sum4/1 -> Product7/2, Product4/2  "Vc"
  Unit Delay5/1 -> Sum4/2
  Sum3/1 -> Gain4/1
  Product3/1 -> Sum3/1
  Product4/1 -> Mux2/1  "Vin"
  Demux/2 -> An_Vbl/1
  Product7/1 -> Mux2/2  "Vbl"
  Unit Delay7/1 -> Product3/2
  An_Ipos/1 -> Mux1/1

== system 20240109_HVDCMMCInterconnection/Sources1/3ph SM1 ==
  Uref_An : Inport
  An_Ipos : Inport  Port=2
  An_Icap : Inport  Port=3
  Demux : Demux  Outputs=2
  Demux2 : Demux  Outputs=2
  Discrete-Time Integrator1 : DiscreteIntegrator  IntegratorMethod=Integration: Trapezoidal  gainval=1  SampleTime=Ts_Power  UpperSaturationLimit=5000  LowerSaturationLimit=500  ICPrevOutput=DiscIntNeverNeededParam  ICPrevScaledInput=DiscIntNeverNeededParam
  Gain1 : Gain  Gain=Nb_PM
  Gain4 : Gain  Gain=1/(C_PM*Nb_PM)
  Gain5 : Gain  Gain=2
  Mux1 : Mux  Inputs=2
  Mux2 : Mux  Inputs=2
  Product3 : Product
  Product4 : Product
  Product7 : Product
  Sum3 : Sum  Inputs=1  InputSameDT=on  SaturateOnIntegerOverflow=on  OutDataTypeStr=Inherit: Same as first input
  Sum4 : Sum  Inputs=+-  InputSameDT=on  SaturateOnIntegerOverflow=on  OutDataTypeStr=Inherit: Same as first input
  Unit Delay5 : UnitDelay  SampleTime=Ts_Power  HasFrameUpgradeWarning=on
  Unit Delay6 : UnitDelay  SampleTime=Ts_Power  HasFrameUpgradeWarning=on
  Unit Delay7 : UnitDelay  SampleTime=Ts_Power  HasFrameUpgradeWarning=on
  An_Vbl : Outport
  An_Vin : Outport  Port=2
  wires:
  Gain5/1 -> Sum4/1
  Gain1/1 -> Demux2/1, Product3/1
  Mux2/1 -> Demux/1
  Demux/1 -> An_Vin/1
  Uref_An/1 -> Gain1/1
  Gain4/1 -> Discrete-Time Integrator1/1
  Mux1/1 -> Unit Delay7/1
  Demux2/2 -> Product7/1
  Unit Delay6/1 -> Gain5/1, Unit Delay5/1
  An_Icap/1 -> Mux1/2
  Demux2/1 -> Product4/1
  Discrete-Time Integrator1/1 -> Unit Delay6/1
  Sum4/1 -> Product7/2, Product4/2  "Vc"
  Unit Delay5/1 -> Sum4/2
  Sum3/1 -> Gain4/1
  Product3/1 -> Sum3/1
  Product4/1 -> Mux2/1  "Vin"
  Demux/2 -> An_Vbl/1
  Product7/1 -> Mux2/2  "Vbl"
  Unit Delay7/1 -> Product3/2
  An_Ipos/1 -> Mux1/1

== system 20240109_HVDCMMCInterconnection/Sources1/3ph SM2 ==
  Uref_An : Inport
  An_Ipos : Inport  Port=2
  An_Icap : Inport  Port=3
  Demux : Demux  Outputs=2
  Demux2 : Demux  Outputs=2
  Discrete-Time Integrator1 : DiscreteIntegrator  IntegratorMethod=Integration: Trapezoidal  gainval=1  SampleTime=Ts_Power  UpperSaturationLimit=5000  LowerSaturationLimit=500  ICPrevOutput=DiscIntNeverNeededParam  ICPrevScaledInput=DiscIntNeverNeededParam
  Gain1 : Gain  Gain=Nb_PM
  Gain4 : Gain  Gain=1/(C_PM*Nb_PM)
  Gain5 : Gain  Gain=2
  Mux1 : Mux  Inputs=2
  Mux2 : Mux  Inputs=2
  Product3 : Product
  Product4 : Product
  Product7 : Product
  Sum3 : Sum  Inputs=1  InputSameDT=on  SaturateOnIntegerOverflow=on  OutDataTypeStr=Inherit: Same as first input
  Sum4 : Sum  Inputs=+-  InputSameDT=on  SaturateOnIntegerOverflow=on  OutDataTypeStr=Inherit: Same as first input
  Unit Delay5 : UnitDelay  SampleTime=Ts_Power  HasFrameUpgradeWarning=on
  Unit Delay6 : UnitDelay  SampleTime=Ts_Power  HasFrameUpgradeWarning=on
  Unit Delay7 : UnitDelay  SampleTime=Ts_Power  HasFrameUpgradeWarning=on
  An_Vbl : Outport
  An_Vin : Outport  Port=2
  wires:
  Gain5/1 -> Sum4/1
  Gain1/1 -> Demux2/1, Product3/1
  Mux2/1 -> Demux/1
  Demux/1 -> An_Vin/1
  Uref_An/1 -> Gain1/1
  Gain4/1 -> Discrete-Time Integrator1/1
  Mux1/1 -> Unit Delay7/1
  Demux2/2 -> Product7/1
  Unit Delay6/1 -> Gain5/1, Unit Delay5/1
  An_Icap/1 -> Mux1/2
  Demux2/1 -> Product4/1
  Discrete-Time Integrator1/1 -> Unit Delay6/1
  Sum4/1 -> Product7/2, Product4/2  "Vc"
  Unit Delay5/1 -> Sum4/2
  Sum3/1 -> Gain4/1
  Product3/1 -> Sum3/1
  Product4/1 -> Mux2/1  "Vin"
  Demux/2 -> An_Vbl/1
  Product7/1 -> Mux2/2  "Vbl"
  Unit Delay7/1 -> Product3/2
  An_Ipos/1 -> Mux1/1

== system 20240109_HVDCMMCInterconnection/Sources1/3ph SM3 ==
  Uref_An : Inport
  An_Ipos : Inport  Port=2
  An_Icap : Inport  Port=3
  Demux : Demux  Outputs=2
  Demux2 : Demux  Outputs=2
  Discrete-Time Integrator1 : DiscreteIntegrator  IntegratorMethod=Integration: Trapezoidal  gainval=1  SampleTime=Ts_Power  UpperSaturationLimit=5000  LowerSaturationLimit=500  ICPrevOutput=DiscIntNeverNeededParam  ICPrevScaledInput=DiscIntNeverNeededParam
  Gain1 : Gain  Gain=Nb_PM
  Gain4 : Gain  Gain=1/(C_PM*Nb_PM)
  Gain5 : Gain  Gain=2
  Mux1 : Mux  Inputs=2
  Mux2 : Mux  Inputs=2
  Product3 : Product
  Product4 : Product
  Product7 : Product
  Sum3 : Sum  Inputs=1  InputSameDT=on  SaturateOnIntegerOverflow=on  OutDataTypeStr=Inherit: Same as first input
  Sum4 : Sum  Inputs=+-  InputSameDT=on  SaturateOnIntegerOverflow=on  OutDataTypeStr=Inherit: Same as first input
  Unit Delay5 : UnitDelay  SampleTime=Ts_Power  HasFrameUpgradeWarning=on
  Unit Delay6 : UnitDelay  SampleTime=Ts_Power  HasFrameUpgradeWarning=on
  Unit Delay7 : UnitDelay  SampleTime=Ts_Power  HasFrameUpgradeWarning=on
  An_Vbl : Outport
  An_Vin : Outport  Port=2
  wires:
  Gain5/1 -> Sum4/1
  Gain1/1 -> Demux2/1, Product3/1
  Mux2/1 -> Demux/1
  Demux/1 -> An_Vin/1
  Uref_An/1 -> Gain1/1
  Gain4/1 -> Discrete-Time Integrator1/1
  Mux1/1 -> Unit Delay7/1
  Demux2/2 -> Product7/1
  Unit Delay6/1 -> Gain5/1, Unit Delay5/1
  An_Icap/1 -> Mux1/2
  Demux2/1 -> Product4/1
  Discrete-Time Integrator1/1 -> Unit Delay6/1
  Sum4/1 -> Product7/2, Product4/2  "Vc"
  Unit Delay5/1 -> Sum4/2
  Sum3/1 -> Gain4/1
  Product3/1 -> Sum3/1
  Product4/1 -> Mux2/1  "Vin"
  Demux/2 -> An_Vbl/1
  Product7/1 -> Mux2/2  "Vbl"
  Unit Delay7/1 -> Product3/2
  An_Ipos/1 -> Mux1/1

== system 20240109_HVDCMMCInterconnection/Sources1/3ph SM4 ==
  Uref_An : Inport
  An_Ipos : Inport  Port=2
  An_Icap : Inport  Port=3
  Demux : Demux  Outputs=2
  Demux2 : Demux  Outputs=2
  Discrete-Time Integrator1 : DiscreteIntegrator  IntegratorMethod=Integration: Trapezoidal  gainval=1  SampleTime=Ts_Power  UpperSaturationLimit=5000  LowerSaturationLimit=500  ICPrevOutput=DiscIntNeverNeededParam  ICPrevScaledInput=DiscIntNeverNeededParam
  Gain1 : Gain  Gain=Nb_PM
  Gain4 : Gain  Gain=1/(C_PM*Nb_PM)
  Gain5 : Gain  Gain=2
  Mux1 : Mux  Inputs=2
  Mux2 : Mux  Inputs=2
  Product3 : Product
  Product4 : Product
  Product7 : Product
  Sum3 : Sum  Inputs=1  InputSameDT=on  SaturateOnIntegerOverflow=on  OutDataTypeStr=Inherit: Same as first input
  Sum4 : Sum  Inputs=+-  InputSameDT=on  SaturateOnIntegerOverflow=on  OutDataTypeStr=Inherit: Same as first input
  Unit Delay5 : UnitDelay  SampleTime=Ts_Power  HasFrameUpgradeWarning=on
  Unit Delay6 : UnitDelay  SampleTime=Ts_Power  HasFrameUpgradeWarning=on
  Unit Delay7 : UnitDelay  SampleTime=Ts_Power  HasFrameUpgradeWarning=on
  An_Vbl : Outport
  An_Vin : Outport  Port=2
  wires:
  Gain5/1 -> Sum4/1
  Gain1/1 -> Demux2/1, Product3/1
  Mux2/1 -> Demux/1
  Demux/1 -> An_Vin/1
  Uref_An/1 -> Gain1/1
  Gain4/1 -> Discrete-Time Integrator1/1
  Mux1/1 -> Unit Delay7/1
  Demux2/2 -> Product7/1
  Unit Delay6/1 -> Gain5/1, Unit Delay5/1
  An_Icap/1 -> Mux1/2
  Demux2/1 -> Product4/1
  Discrete-Time Integrator1/1 -> Unit Delay6/1
  Sum4/1 -> Product7/2, Product4/2  "Vc"
  Unit Delay5/1 -> Sum4/2
  Sum3/1 -> Gain4/1
  Product3/1 -> Sum3/1
  Product4/1 -> Mux2/1  "Vin"
  Demux/2 -> An_Vbl/1
  Product7/1 -> Mux2/2  "Vbl"
  Unit Delay7/1 -> Product3/2
  An_Ipos/1 -> Mux1/1

== system 20240109_HVDCMMCInterconnection/Sources1/3ph SM5 ==
  Uref_An : Inport
  An_Ipos : Inport  Port=2
  An_Icap : Inport  Port=3
  Demux : Demux  Outputs=2
  Demux2 : Demux  Outputs=2
  Discrete-Time Integrator1 : DiscreteIntegrator  IntegratorMethod=Integration: Trapezoidal  gainval=1  SampleTime=Ts_Power  UpperSaturationLimit=5000  LowerSaturationLimit=500  ICPrevOutput=DiscIntNeverNeededParam  ICPrevScaledInput=DiscIntNeverNeededParam
  Gain1 : Gain  Gain=Nb_PM
  Gain4 : Gain  Gain=1/(C_PM*Nb_PM)
  Gain5 : Gain  Gain=2
  Mux1 : Mux  Inputs=2
  Mux2 : Mux  Inputs=2
  Product3 : Product
  Product4 : Product
  Product7 : Product
  Sum3 : Sum  Inputs=1  InputSameDT=on  SaturateOnIntegerOverflow=on  OutDataTypeStr=Inherit: Same as first input
  Sum4 : Sum  Inputs=+-  InputSameDT=on  SaturateOnIntegerOverflow=on  OutDataTypeStr=Inherit: Same as first input
  Unit Delay5 : UnitDelay  SampleTime=Ts_Power  HasFrameUpgradeWarning=on
  Unit Delay6 : UnitDelay  SampleTime=Ts_Power  HasFrameUpgradeWarning=on
  Unit Delay7 : UnitDelay  SampleTime=Ts_Power  HasFrameUpgradeWarning=on
  An_Vbl : Outport
  An_Vin : Outport  Port=2
  wires:
  Gain5/1 -> Sum4/1
  Gain1/1 -> Demux2/1, Product3/1
  Mux2/1 -> Demux/1
  Demux/1 -> An_Vin/1
  Uref_An/1 -> Gain1/1
  Gain4/1 -> Discrete-Time Integrator1/1
  Mux1/1 -> Unit Delay7/1
  Demux2/2 -> Product7/1
  Unit Delay6/1 -> Gain5/1, Unit Delay5/1
  An_Icap/1 -> Mux1/2
  Demux2/1 -> Product4/1
  Discrete-Time Integrator1/1 -> Unit Delay6/1
  Sum4/1 -> Product7/2, Product4/2  "Vc"
  Unit Delay5/1 -> Sum4/2
  Sum3/1 -> Gain4/1
  Product3/1 -> Sum3/1
  Product4/1 -> Mux2/1  "Vin"
  Demux/2 -> An_Vbl/1
  Product7/1 -> Mux2/2  "Vbl"
  Unit Delay7/1 -> Product3/2
  An_Ipos/1 -> Mux1/1

== system 20240109_HVDCMMCInterconnection/Sources1/3ph SM6 ==
  Uref_An : Inport
  An_Ipos : Inport  Port=2
  An_Icap : Inport  Port=3
  Demux : Demux  Outputs=2
  Demux2 : Demux  Outputs=2
  Discrete-Time Integrator1 : DiscreteIntegrator  IntegratorMethod=Integration: Trapezoidal  gainval=1  SampleTime=Ts_Power  UpperSaturationLimit=5000  LowerSaturationLimit=500  ICPrevOutput=DiscIntNeverNeededParam  ICPrevScaledInput=DiscIntNeverNeededParam
  Gain1 : Gain  Gain=Nb_PM
  Gain4 : Gain  Gain=1/(C_PM*Nb_PM)
  Gain5 : Gain  Gain=2
  Mux1 : Mux  Inputs=2
  Mux2 : Mux  Inputs=2
  Product3 : Product
  Product4 : Product
  Product7 : Product
  Sum3 : Sum  Inputs=1  InputSameDT=on  SaturateOnIntegerOverflow=on  OutDataTypeStr=Inherit: Same as first input
  Sum4 : Sum  Inputs=+-  InputSameDT=on  SaturateOnIntegerOverflow=on  OutDataTypeStr=Inherit: Same as first input
  Unit Delay5 : UnitDelay  SampleTime=Ts_Power  HasFrameUpgradeWarning=on
  Unit Delay6 : UnitDelay  SampleTime=Ts_Power  HasFrameUpgradeWarning=on
  Unit Delay7 : UnitDelay  SampleTime=Ts_Power  HasFrameUpgradeWarning=on
  An_Vbl : Outport
  An_Vin : Outport  Port=2
  wires:
  Gain5/1 -> Sum4/1
  Gain1/1 -> Demux2/1, Product3/1
  Mux2/1 -> Demux/1
  Demux/1 -> An_Vin/1
  Uref_An/1 -> Gain1/1
  Gain4/1 -> Discrete-Time Integrator1/1
  Mux1/1 -> Unit Delay7/1
  Demux2/2 -> Product7/1
  Unit Delay6/1 -> Gain5/1, Unit Delay5/1
  An_Icap/1 -> Mux1/2
  Demux2/1 -> Product4/1
  Discrete-Time Integrator1/1 -> Unit Delay6/1
  Sum4/1 -> Product7/2, Product4/2  "Vc"
  Unit Delay5/1 -> Sum4/2
  Sum3/1 -> Gain4/1
  Product3/1 -> Sum3/1
  Product4/1 -> Mux2/1  "Vin"
  Demux/2 -> An_Vbl/1
  Product7/1 -> Mux2/2  "Vbl"
  Unit Delay7/1 -> Product3/2
  An_Ipos/1 -> Mux1/1

== system 20240109_HVDCMMCInterconnection/Subsystem/3ph SM9 ==
  Uref_An : Inport
  An_Ipos : Inport  Port=2
  An_Icap : Inport  Port=3
  Demux : Demux  Outputs=2
  Demux2 : Demux  Outputs=2
  Discrete-Time Integrator1 : DiscreteIntegrator  IntegratorMethod=Integration: Trapezoidal  gainval=1  SampleTime=Ts_Power  UpperSaturationLimit=5000  LowerSaturationLimit=500  ICPrevOutput=DiscIntNeverNeededParam  ICPrevScaledInput=DiscIntNeverNeededParam
  Gain1 : Gain  Gain=Nb_PM
  Gain4 : Gain  Gain=1/(C_PM*Nb_PM)
  Gain5 : Gain  Gain=2
  Mux1 : Mux  Inputs=2
  Mux2 : Mux  Inputs=2
  Product3 : Product
  Product4 : Product
  Product7 : Product
  Sum3 : Sum  Inputs=1  InputSameDT=on  SaturateOnIntegerOverflow=on  OutDataTypeStr=Inherit: Same as first input
  Sum4 : Sum  Inputs=+-  InputSameDT=on  SaturateOnIntegerOverflow=on  OutDataTypeStr=Inherit: Same as first input
  Unit Delay5 : UnitDelay  SampleTime=Ts_Power  HasFrameUpgradeWarning=on
  Unit Delay6 : UnitDelay  SampleTime=Ts_Power  HasFrameUpgradeWarning=on
  Unit Delay7 : UnitDelay  SampleTime=Ts_Power  HasFrameUpgradeWarning=on
  An_Vbl : Outport
  An_Vin : Outport  Port=2
  wires:
  An_Ipos/1 -> Mux1/1
  Unit Delay7/1 -> Product3/2
  Product7/1 -> Mux2/2  "Vbl"
  Demux/2 -> An_Vbl/1
  Product4/1 -> Mux2/1  "Vin"
  Product3/1 -> Sum3/1
  Sum3/1 -> Gain4/1
  Unit Delay5/1 -> Sum4/2
  Sum4/1 -> Product4/2, Product7/2  "Vc"
  Discrete-Time Integrator1/1 -> Unit Delay6/1
  Demux2/1 -> Product4/1
  An_Icap/1 -> Mux1/2
  Unit Delay6/1 -> Unit Delay5/1, Gain5/1
  Demux2/2 -> Product7/1
  Mux1/1 -> Unit Delay7/1
  Gain4/1 -> Discrete-Time Integrator1/1
  Uref_An/1 -> Gain1/1
  Demux/1 -> An_Vin/1
  Mux2/1 -> Demux/1
  Gain1/1 -> Product3/1, Demux2/1
  Gain5/1 -> Sum4/1

== system 20240109_HVDCMMCInterconnection/Subsystem/SW_ON ==
  In1 : Inport
  SW : Inport  Port=2
  Compare To Constant3 : simulink/Logic and Bit Operations/Compare To Constant  relop=>  const=0.5  OutDataTypeStr=boolean
  Constant : Constant  Value=0
  Gain : Gain  Gain=1./D_R  SaturateOnIntegerOverflow=on  OutDataTypeStr=Inherit: Same as input  ParamDataTypeStr=Inherit: Same as input
  Mux21 : Mux  Inputs=2
  NOT : Logic  Operator=NOT  IconShape=distinctive  AllPortsSameDT=off  OutDataTypeStr=boolean
  Product6 : Product
  Product7 : Product
  Saturation : Saturate  UpperLimit=inf  LowerLimit=0
  Sum5 : Sum  Inputs=1  InputSameDT=on  SaturateOnIntegerOverflow=on  OutDataTypeStr=Inherit: Same as first input
  Out1 : Outport
  wires:
  Saturation/1 -> Out1/1
  Gain/1 -> Product7/1
  Constant/1 -> Product6/2
  Compare To Constant3/1 -> NOT/1, Product7/2
  Product7/1 -> Mux21/1
  SW/1 -> Compare To Constant3/1
  In1/1 -> Gain/1
  NOT/1 -> Product6/1
  Product6/1 -> Mux21/2
  Mux21/1 -> Sum5/1
  Sum5/1 -> Saturation/1

== system 20240109_HVDCMMCInterconnection/Subsystem/SW_ON1 ==
  In1 : Inport
  SW : Inport  Port=2
  Compare To Constant3 : simulink/Logic and Bit Operations/Compare To Constant  relop=>  const=0.5  OutDataTypeStr=boolean
  Constant : Constant  Value=0
  Gain : Gain  Gain=1./D_R  SaturateOnIntegerOverflow=on  OutDataTypeStr=Inherit: Same as input  ParamDataTypeStr=Inherit: Same as input
  Mux21 : Mux  Inputs=2
  NOT : Logic  Operator=NOT  IconShape=distinctive  AllPortsSameDT=off  OutDataTypeStr=boolean
  Product6 : Product
  Product7 : Product
  Saturation : Saturate  UpperLimit=inf  LowerLimit=0
  Sum5 : Sum  Inputs=1  InputSameDT=on  SaturateOnIntegerOverflow=on  OutDataTypeStr=Inherit: Same as first input
  Out1 : Outport
  wires:
  Saturation/1 -> Out1/1
  Gain/1 -> Product7/1
  Constant/1 -> Product6/2
  Compare To Constant3/1 -> NOT/1, Product7/2
  Product7/1 -> Mux21/1
  SW/1 -> Compare To Constant3/1
  In1/1 -> Gain/1
  NOT/1 -> Product6/1
  Product6/1 -> Mux21/2
  Mux21/1 -> Sum5/1
  Sum5/1 -> Saturation/1

== system 20240109_HVDCMMCInterconnection/Subsystem/Subsystem1 ==
  Uswitch : Inport
  status : Inport  Port=2
  0 1 : Constant  Value=0
  Gain : Gain  Gain=1./D_R  SaturateOnIntegerOverflow=on  OutDataTypeStr=Inherit: Same as input  ParamDataTypeStr=Inherit: Same as input
  Saturation : Saturate  UpperLimit=inf  LowerLimit=0
  Switch : Switch  Threshold=0.5  SaturateOnIntegerOverflow=off
  iSwitch : Outport
  wires:
  Uswitch/1 -> Gain/1
  Saturation/1 -> iSwitch/1
  Switch/1 -> Saturation/1
  Gain/1 -> Switch/1
  0 1/1 -> Switch/3
  status/1 -> Switch/2
